simulink model "automata_learning"  (R2018a)
settings: Solver=FixedStepAuto  StartTime=0.0  StopTime=T  FixedStep=Ts  RelTol=1e-3
settings Model: Creator=xiaodong  LastModifiedBy=xiaodong

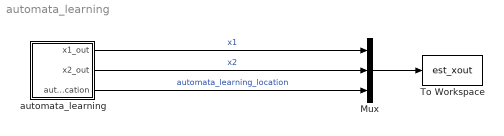
== system automata_learning ==
  Mux : Mux  Inputs=3
  To Workspace : ToWorkspace  VariableName=est_xout  SampleTime=-1
  automata_learning : Stateflow chart  TreatAsAtomicUnit=on
  wires:
  automata_learning/1(x1_out) -> Mux/1  "x1"
  automata_learning/2(x2_out) -> Mux/2  "x2"
  automata_learning/3(automata_learning_location) -> Mux/3  "automata_learning_location"
  Mux/1 -> To Workspace/1

== stateflow chart automata_learning/automata_learning ==
  settings: updateMethod=CONTINUOUS
  state loc1
    du:
    x1_dot = 19.82730190496659 * x1 - 483.35486798081547 * x2 + 6484.962363272905;
    x2_dot = 290.77148099895567 * x1 - 123.04878845950589 * x2 + 1317.1628625802696;
    x1_out=x1;
    x2_out=x2;
    automata_learning_location =1;
  state loc2
    du:
    x1_dot = 9064.579930633307 - 378.81976657547057 * x2 - 271.94735317956656 * x1;
    x2_dot = 452.66677063703537 * x1 - 51.243269544211216 * x2 + 60.72636410524137;
    x1_out=x1;
    x2_out=x2;
    automata_learning_location =2;
  state loc3
    du:
    x1_dot = -196.2833062261343 * x1 - 375.63914385344833 * x2 - 22.514045030926354;
    x2_dot = 456.52232484333217 * x1 - 54.72674559045117 * x2 + 104.7049718555063;
    x1_out=x1;
    x2_out=x2;
    automata_learning_location =3;
  loc3 -> loc1 : [-11.2 * x1 - 0.07218 * x2 + 1.0 > 0.0]
  loc1 -> loc2 : [0.001078 * x1 - 0.08408 * x2 + 1.0 > 0.0]
  (default) -> loc1 : {x1 = x_init(1);
      | x2 = x_init(2);}
  loc2 -> loc3 : [0.0008946 * x1 - 0.08262 * x2 + 1.0 < 0.0]
  data: x1_out output; x1 local; x2_out output; x2 local; automata_learning_location output; x_init constant double size=2 =x_init
  data x1 settings: updateMethod=SF_CONTINUOUS_TIME_DATA
  data x2 settings: updateMethod=SF_CONTINUOUS_TIME_DATA
